simulink model "generic_src"  (Simulink 10.3)
settings: Solver=ode45  StartTime=0.0  StopTime=inf  RelTol=1e-3  EnableMultiTasking=on
undefined symbols (not defined in the file or in its folder): Area_Front, Area_Rear, ay_max_off, ay_max_on, ay_per_mu_max_off, ay_per_mu_max_on, Brake_ratio, brake_valve_ctrl_kP, cat1mode1_higher, cat1mode1_lower, cat1mode2_higher, cat1mode2_lower, cat1mode3_higher, cat1mode3_lower, cat2mode1_higher, cat2mode1_lower, cat2mode2_higher, cat2mode2_lower, cat2mode3_higher, cat2mode3_lower, delta_vel, diff_lock_fac, diff_lock_off, diff_lock_on, ESP_ctrl_kD, ESP_ctrl_kI, ESP_ctrl_kP, ESP_ctrl_restore_kI, ESP_min_throttle_fac, f_ax, f_slip, g, higherlimit_highvel, higherlimit_lowvel, highervel_fac, highervelocity_fac, InitialConditionForIntegrator, limit_acc, limit_selectlow, limit_starting, limit_vdiff, locktime_throttle, lowerlimit_highvel, lowerlimit_lowvel, lowervel_fac, lowervelocity_fac, min_throttle, MPS2KMPH, MSR_ctrl_kD, MSR_ctrl_kI, MSR_ctrl_kP, MSR_min_throttle_fac, PID_kP_sideslip, PID_kP_yawrate, RADpS2RpM, rBrake, RpM2RADpS, SH_SL_switch, sideslip_vel_corr, sidesplip_deviation_max ... (+35)
libraries: CarMaker4SL x137, simulink x57, simulink_extras x6
(part 4 of 12)

== system generic_src/CarMaker/IPG Vehicle/Brake/HydBrakeCU Example/ESP Controller/ESP Input Signals ==
  HydBrakeCtrl_In : Inport
  " " : simulink_extras/Transformations/Radians to Degrees
  "   " : simulink_extras/Transformations/Radians to Degrees
  Bus Creator1 : BusCreator  Inputs=20
  Bus Selector : BusSelector  OutputSignals=Omega_B z,Acc_B y,Acc_B x
  Bus Selector1 : BusSelector  OutputSignals=HydBrakeCU pMC,HydBrakeCU pWB_FL,HydBrakeCU pWB_FR,HydBrakeCU pWB_RL,HydBrakeCU pWB_RR,HydBrakeCU Park,HydBrakeCU Pedal
  Car InertialSensor : CarMaker4SL/Sensors/Inertial Sensor  xname=YRS  xstime=Continuous
  Gain{,6,9..10,12..17} (10 alike) : Gain  SaturateOnIntegerOverflow=on  OutDataTypeStr=Inherit: Same as input  ParamDataTypeStr=Inherit: Same as input
  Gain{1..5,11} (6 alike) : Gain  Gain=RADpS2RpM  SaturateOnIntegerOverflow=on  OutDataTypeStr=Inherit: Same as input  ParamDataTypeStr=Inherit: Same as input
  Gain7 : Gain  Gain=1/g  SaturateOnIntegerOverflow=on  OutDataTypeStr=Inherit: Same as input  ParamDataTypeStr=Inherit: Same as input
  Gain8 : Gain  Gain=1/g  SaturateOnIntegerOverflow=on  OutDataTypeStr=Inherit: Same as input  ParamDataTypeStr=Inherit: Same as input
  Read CM Dict1 : CarMaker4SL/Read CM Dict  xname=Car.WheelSpd_FL  xsync=off  xstime=Continuous
  Read CM Dict10 : CarMaker4SL/Read CM Dict  xname=PT.Clutch.0.rotv_out  xsync=off  xstime=Continuous
  Read CM Dict11 : CarMaker4SL/Read CM Dict  xname=Steer.WhlAng  xsync=off  xstime=Continuous
  Read CM Dict12 : CarMaker4SL/Read CM Dict  xname=PT.Engine.Trq  xsync=off  xstime=Continuous
  Read CM Dict15 : CarMaker4SL/Read CM Dict  xname=PT.GearBox.GearNo  xsync=off  xstime=Continuous
  Read CM Dict2 : CarMaker4SL/Read CM Dict  xname=Car.WheelSpd_FR  xsync=off  xstime=Continuous
  Read CM Dict3 : CarMaker4SL/Read CM Dict  xname=Car.WheelSpd_RL  xsync=off  xstime=Continuous
  Read CM Dict4 : CarMaker4SL/Read CM Dict  xname=Car.WheelSpd_RR  xsync=off  xstime=Continuous
  Read CM Dict7 : CarMaker4SL/Read CM Dict  xname=PT.Engine.rotv  xsync=off  xstime=Continuous
  Read CM Dict9 : CarMaker4SL/Read CM Dict  xname=VC.Gas  xsync=off  xstime=Continuous
  Terminator : Terminator
  ESP Signals : Outport  VectorParamsAs1DForOutWhenUnconnected=off
  wires:
  Gain9/1 -> Bus Creator1/9  "Engine crankshaft output torque [Nm]"
  Gain13/1 -> Bus Creator1/14  "GearState [-]"
  " "/1 -> Bus Creator1/13  "Steering Wheel Angle [deg]"
  Gain11/1 -> Bus Creator1/12  "Torque Converter Speed [rpm]"
  Gain10/1 -> Bus Creator1/10  "Master Cylinder Pressure [bar]"
  Gain8/1 -> Bus Creator1/7  "Sensor Longitudinal acceleration [g]"
  Gain7/1 -> Bus Creator1/6  "Sensor Lateral acceleration [g]"
  "   "/1 -> Bus Creator1/5  "Sensor YawRate [degs]"
  Gain4/1 -> Bus Creator1/4  "WheelSpd RR [rpm]"
  Gain5/1 -> Bus Creator1/3  "WheelSpd RL [rpm]"
  Gain3/1 -> Bus Creator1/2  "WheelSpd FR [rpm]"
  Gain2/1 -> Bus Creator1/1  "WheelSpd FL [rpm]"
  Read CM Dict15/1 -> Gain13/1  "GearNumber [-]"
  Gain1/1 -> Bus Creator1/8  "Engine Speed [rpm]"
  Bus Selector/1 -> "   "/1  "<Omega_B z>"
  Bus Selector/3 -> Gain8/1  "<Acc_B x>"
  Car InertialSensor/2 -> Bus Selector/1
  Read CM Dict11/1 -> " "/1  "Steering Angle [rad]"
  Read CM Dict10/1 -> Gain11/1  "Clucth OutShaft [rad/s]"
  Read CM Dict9/1 -> Gain/1  "Accelerator pedal [-]"
  Bus Selector1/1 -> Gain10/1  "<HydBrakeCU pMC>"
  Read CM Dict1/1 -> Gain2/1  "WheelSpd FL [rad]/s]"
  Read CM Dict2/1 -> Gain3/1  "WheelSpd FR [rad/s]"
  Read CM Dict3/1 -> Gain5/1  "WheelSpd RL [rad/s]"
  Bus Selector/2 -> Gain7/1  "<Acc_B y>"
  Read CM Dict4/1 -> Gain4/1  "WheelSpd RR [rad/s]"
  Gain/1 -> Bus Creator1/11  "Throttle Valve Position"
  Read CM Dict12/1 -> Gain9/1  "Engine Torque [Nm]"
  Read CM Dict7/1 -> Gain1/1  "Engine RotVel [rad/s]"
  Bus Creator1/1 -> ESP Signals/1
  Bus Selector1/5 -> Gain15/1  "<HydBrakeCU pWB_RR>"
  Bus Selector1/4 -> Gain14/1  "<HydBrakeCU pWB_RL>"
  Bus Selector1/3 -> Gain12/1  "<HydBrakeCU pWB_FR>"
  Bus Selector1/2 -> Gain6/1  "<HydBrakeCU pWB_FL>"
  Gain6/1 -> Bus Creator1/15  "Cylinder Pressure FL [bar]"
  Gain12/1 -> Bus Creator1/16  "Cylinder Pressure FR [bar]"
  Gain14/1 -> Bus Creator1/17  "Cylinder Pressure RL [bar]"
  Gain15/1 -> Bus Creator1/18  "Cylinder Pressure RR [bar]"
  HydBrakeCtrl_In/1 -> Bus Selector1/1
  Car InertialSensor/1 -> Terminator/1
  Bus Selector1/6 -> Gain16/1  "<HydBrakeCU Park>"
  Gain16/1 -> Bus Creator1/19  "Park Brake Position"
  Bus Selector1/7 -> Gain17/1  "<HydBrakeCU Pedal>"
  Gain17/1 -> Bus Creator1/20  "Brake Pedal Position"

== system generic_src/CarMaker/IPG Vehicle/Brake/HydBrakeCU Example/ESP Controller/Ideal Input Signals ==
  Bus Creator1 : BusCreator  Inputs=8
  Bus Creator2 : BusCreator  Inputs=4
  Bus Creator3 : BusCreator  Inputs=2
  Bus Creator4 : BusCreator  Inputs=2
  Bus Creator5 : BusCreator  Inputs=3
  Bus Creator6 : BusCreator  Inputs=2
  Read CM Dict1 : CarMaker4SL/Read CM Dict  xname=Car.Pitch  xsync=off  xstime=Continuous
  Read CM Dict10 : CarMaker4SL/Read CM Dict  xname=Car.FzRL  xsync=off  xstime=Continuous
  Read CM Dict11 : CarMaker4SL/Read CM Dict  xname=Car.YawRate  xsync=off  xstime=Continuous
  Read CM Dict13 : CarMaker4SL/Read CM Dict  xname=Car.CRL.Trq_T2W  xsync=off  xstime=Continuous
  Read CM Dict14 : CarMaker4SL/Read CM Dict  xname=Car.LongSlipRL  xsync=off  xstime=Continuous
  Read CM Dict16 : CarMaker4SL/Read CM Dict  xname=Car.CRR.Trq_T2W  xsync=off  xstime=Continuous
  Read CM Dict17 : CarMaker4SL/Read CM Dict  xname=Car.FzRR  xsync=off  xstime=Continuous
  Read CM Dict19 : CarMaker4SL/Read CM Dict  xname=Car.LongSlipRR  xsync=off  xstime=Continuous
  Read CM Dict2 : CarMaker4SL/Read CM Dict  xname=Car.v  xsync=off  xstime=Continuous
  Read CM Dict3 : CarMaker4SL/Read CM Dict  xname=Car.muRoadFR  xsync=off  xstime=Continuous
  Read CM Dict4 : CarMaker4SL/Read CM Dict  xname=Car.muRoadRL  xsync=off  xstime=Continuous
  Read CM Dict5 : CarMaker4SL/Read CM Dict  xname=Car.SideSlipAngle  xsync=off  xstime=Continuous
  Read CM Dict6 : CarMaker4SL/Read CM Dict  xname=Car.muRoadFL  xsync=off  xstime=Continuous
  Read CM Dict7 : CarMaker4SL/Read CM Dict  xname=Car.muRoadRR  xsync=off  xstime=Continuous
  Read CM Dict8 : CarMaker4SL/Read CM Dict  xname=Car.vx  xsync=off  xstime=Continuous
  Read CM Dict9 : CarMaker4SL/Read CM Dict  xname=Car.vy  xsync=off  xstime=Continuous
  Ideal_In : Outport  VectorParamsAs1DForOutWhenUnconnected=off
  wires:
  Read CM Dict17/1 -> Bus Creator4/2  "Ideal_FzRR"
  Read CM Dict10/1 -> Bus Creator4/1  "Ideal_FzRL"
  Read CM Dict16/1 -> Bus Creator3/2  "Ideal_Trq2WRR"
  Read CM Dict13/1 -> Bus Creator3/1  "Ideal_Trq2WRL"
  Read CM Dict6/1 -> Bus Creator2/1  "Ideal_muFL"
  Read CM Dict3/1 -> Bus Creator2/2  "Ideal_muFR"
  Read CM Dict4/1 -> Bus Creator2/3  "Ideal_muRL"
  Read CM Dict7/1 -> Bus Creator2/4  "Ideal_muRR"
  Bus Creator1/1 -> Ideal_In/1
  Read CM Dict1/1 -> Bus Creator1/1  "Ideal_Pitch"
  Read CM Dict5/1 -> Bus Creator1/3  "Ideal_SideSlipAngle"
  Read CM Dict2/1 -> Bus Creator5/1  "Ideal_Velocity"
  Read CM Dict8/1 -> Bus Creator5/2  "Ideal_Velocity_x"
  Bus Creator5/1 -> Bus Creator1/2  "Ideal_Velocity"
  Read CM Dict9/1 -> Bus Creator5/3  "Ideal_Velocity_y"
  Read CM Dict14/1 -> Bus Creator6/1  "Ideal_SlipRL"
  Read CM Dict19/1 -> Bus Creator6/2  "Ideal_SlipRR"
  Read CM Dict11/1 -> Bus Creator1/4  "Ideal_YawRate"
  Bus Creator2/1 -> Bus Creator1/5  "Ideal_mu"
  Bus Creator3/1 -> Bus Creator1/6  "Idea_Trq2W"
  Bus Creator4/1 -> Bus Creator1/7  "Ideal_Fz"
  Bus Creator6/1 -> Bus Creator1/8  "Ideal_Slip"

== system generic_src/CarMaker/IPG Vehicle/Brake/HydBrakeCU Example/ESP Controller/Output Signals ESP ==
  ESP Out : Inport
  Bus Creator : BusCreator  Inputs=6
  Bus Selector : BusSelector  OutputSignals=ECU Flags,Brake Valves,Pilot Valves,Suction Valves,Pump Ctrl,VC_Out.BrakePark,VC_Out.Brake Pedal Position,Diff_Torque,VC_Out.Load_lim
  Bus Selector1 : BusSelector  OutputSignals=ESP On,ASR On,ABS On,HSA On
  Bus Selector2 : BusSelector  OutputSignals=ASR On,MSR On,BMR On
  Bus Selector4 : BusSelector  OutputSignals=FrontDiff_Torque
  Data Type Conversion : DataTypeConversion
  Define CM Dict1 : CarMaker4SL/Define CM Dict  xname=ESP.ASR.MSR.active  xmono=off  xtype=Char  xdvaplace=VC  xnstates=2  xfirststate=0  xinitial=0
  Define CM Dict10 : CarMaker4SL/Define CM Dict  xname=ESP.ESP.active  xmono=off  xtype=Char  xdvaplace=VC  xnstates=2  xfirststate=0  xinitial=0
  Define CM Dict2 : CarMaker4SL/Define CM Dict  xname=ESP.ASR.BMR.active  xmono=off  xtype=Char  xdvaplace=VC  xnstates=2  xfirststate=0  xinitial=0
  Define CM Dict3 : CarMaker4SL/Define CM Dict  xname=ESP.ASR.active  xmono=off  xtype=Char  xdvaplace=VC  xnstates=2  xfirststate=0  xinitial=0
  Define CM Dict4 : CarMaker4SL/Define CM Dict  xname=ESP.HSA.active  xmono=off  xtype=Char  xdvaplace=VC  xnstates=2  xfirststate=0  xinitial=0
  Define CM Dict6 : CarMaker4SL/Define CM Dict  xname=ESP.ESP.lamp  xmono=off  xtype=Char  xdvaplace=VC  xnstates=2  xfirststate=0  xinitial=0
  Define CM Dict9 : CarMaker4SL/Define CM Dict  xname=ESP.ABS.Active  xmono=off  xtype=Char  xdvaplace=VC  xnstates=2  xfirststate=0  xinitial=0
  Logical Operator : Logic  Operator=OR  AllPortsSameDT=off  OutDataTypeStr=boolean
  Read CM Dict3 : CarMaker4SL/Read CM Dict  xname=ESP.User.ESP_off  xsync=off  xstime=Continuous
  Write CM Dict : CarMaker4SL/Write CM Dict  xname=PT.ECU.Load_lim_max  xsync=off
  Write CM Dict12 : CarMaker4SL/Write CM Dict  xname=ESP.ASR.MSR.active  xsync=off
  Write CM Dict13 : CarMaker4SL/Write CM Dict  xname=ESP.ASR.BMR.active  xsync=off
  Write CM Dict15 : CarMaker4SL/Write CM Dict  xname=ESP.ASR.active  xsync=off
  Write CM Dict17 : CarMaker4SL/Write CM Dict  xname=ESP.ABS.Active  xsync=off
  Write CM Dict18 : CarMaker4SL/Write CM Dict  xname=ESP.ESP.active  xsync=off
  Write CM Dict19 : CarMaker4SL/Write CM Dict  xname=PT.Gen.DL.FDiff.DVA.Trq_A2B  xsync=off
  Write CM Dict20 : CarMaker4SL/Write CM Dict  xname=ESP.HSA.active  xsync=off
  Write CM Dict21 : CarMaker4SL/Write CM Dict  xname=ESP.ESP.lamp  xsync=off
  HydBrakeCU_Out : Outport  VectorParamsAs1DForOutWhenUnconnected=off
  wires:
  ESP Out/1 -> Bus Selector/1
  Bus Selector/1 -> Bus Selector1/1  "<ECU Flags>"
  Bus Selector1/2 -> Bus Selector2/1  "<ASR On>"
  Bus Selector1/1 -> Logical Operator/2, Write CM Dict18/1  "<ESP On>"
  Bus Selector1/3 -> Write CM Dict17/1  "<ABS On>"
  Bus Selector2/1 -> Write CM Dict15/1  "<ASR On>"
  Bus Selector2/2 -> Write CM Dict12/1  "<MSR On>"
  Bus Selector2/3 -> Write CM Dict13/1  "<BMR On>"
  Bus Selector4/1 -> Write CM Dict19/1  "<FrontDiff_Torque>"
  Bus Selector/8 -> Bus Selector4/1  "<Diff_Torque>"
  Bus Selector1/4 -> Write CM Dict20/1  "<HSA On>"
  Logical Operator/1 -> Data Type Conversion/1
  Read CM Dict3/1 -> Logical Operator/1
  Data Type Conversion/1 -> Write CM Dict21/1
  Bus Selector/2 -> Bus Creator/1  "<Brake Valves>"
  Bus Selector/3 -> Bus Creator/2  "<Pilot Valves>"
  Bus Selector/4 -> Bus Creator/3  "<Suction Valves>"
  Bus Selector/5 -> Bus Creator/4  "<Pump Ctrl>"
  Bus Creator/1 -> HydBrakeCU_Out/1
  Bus Selector/6 -> Bus Creator/5  "<BrakePark>"
  Bus Selector/9 -> Write CM Dict/1  "<Load_lim>"
  Bus Selector/7 -> Bus Creator/6  "<Brake Pedal Position>"

== system generic_src/CarMaker/IPG Vehicle/Brake/HydBrakeCU Example/ESP Controller/User Input Signals1 ==
  note: User_Drive: 1 = Front; 2 = Rear; 3 = AllWheel
  Bus Creator1 : BusCreator  Inputs=5
  Bus Creator2 : BusCreator  Inputs=5
  Bus Creator3 : BusCreator  Inputs=2
  Bus Creator4 : BusCreator  Inputs=2
  Define CM Dict1 : CarMaker4SL/Define CM Dict  xname=ESP.User.ESP_off  xmono=off  xtype=Char  xdvaplace=IO_Out  xnstates=2  xfirststate=0  xinitial=0
  Define CM Dict10 : CarMaker4SL/Define CM Dict  xname=ESP.User.HSA_off  xmono=off  xtype=Char  xdvaplace=IO_Out  xnstates=2  xfirststate=0  xinitial=0
  Define CM Dict11 : CarMaker4SL/Define CM Dict  xname=ESP.User.oneWheel_on  xmono=off  xtype=Char  xdvaplace=IO_Out  xnstates=2  xfirststate=0  xinitial=0
  Define CM Dict2 : CarMaker4SL/Define CM Dict  xname=ESP.User.ASR_off  xmono=off  xtype=Char  xdvaplace=IO_Out  xnstates=2  xfirststate=0  xinitial=0
  Define CM Dict3 : CarMaker4SL/Define CM Dict  xname=ESP.User.ABS_off  xmono=off  xtype=Char  xdvaplace=IO_Out  xnstates=2  xfirststate=0  xinitial=0
  Define CM Dict4 : CarMaker4SL/Define CM Dict  xname=ESP.User.ESP_all_off  xmono=off  xtype=Char  xdvaplace=IO_Out  xnstates=2  xfirststate=0  xinitial=0
  Define CM Dict5 : CarMaker4SL/Define CM Dict  xname=ESP.User.Drive  xmono=off  xtype=Char  xdvaplace=IO_Out  xnstates=3  xfirststate=1  xinitial=1
  Define CM Dict6 : CarMaker4SL/Define CM Dict  xname=ESP.User.SideSlip_estimator_on  xmono=off  xtype=Char  xdvaplace=IO_Out  xnstates=2  xfirststate=0  xinitial=0
  Define CM Dict7 : CarMaker4SL/Define CM Dict  xname=ESP.User.mue_estimator_on  xmono=off  xtype=Char  xdvaplace=IO_Out  xnstates=2  xfirststate=0  xinitial=0
  Define CM Dict8 : CarMaker4SL/Define CM Dict  xname=ESP.User.DiffLockDVA_on  xmono=off  xtype=Char  xdvaplace=IO_Out  xnstates=2  xfirststate=0  xinitial=0
  Define CM Dict9 : CarMaker4SL/Define CM Dict  xname=ESP.User.DiffLockDVA_Trq  xunit=Nm  xmono=off  xtype=Double4  xdvaplace=IO_Out  xnstates=2  xfirststate=0  xinitial=0
  Read CM Dict1 : CarMaker4SL/Read CM Dict  xname=ESP.User.Drive  xsync=off  xstime=Continuous
  Read CM Dict10 : CarMaker4SL/Read CM Dict  xname=ESP.User.HSA_off  xsync=off  xstime=Continuous
  Read CM Dict11 : CarMaker4SL/Read CM Dict  xname=ESP.User.oneWheel_on  xsync=off  xstime=Continuous
  Read CM Dict2 : CarMaker4SL/Read CM Dict  xname=ESP.User.ESP_all_off  xsync=off  xstime=Continuous
  Read CM Dict3 : CarMaker4SL/Read CM Dict  xname=ESP.User.ESP_off  xsync=off  xstime=Continuous
  Read CM Dict4 : CarMaker4SL/Read CM Dict  xname=ESP.User.ASR_off  xsync=off  xstime=Continuous
  Read CM Dict5 : CarMaker4SL/Read CM Dict  xname=ESP.User.ABS_off  xsync=off  xstime=Continuous
  Read CM Dict6 : CarMaker4SL/Read CM Dict  xname=ESP.User.SideSlip_estimator_on  xsync=off  xstime=Continuous
  Read CM Dict7 : CarMaker4SL/Read CM Dict  xname=ESP.User.mue_estimator_on  xsync=off  xstime=Continuous
  Read CM Dict8 : CarMaker4SL/Read CM Dict  xname=ESP.User.DiffLockDVA_on  xsync=off  xstime=Continuous
  Read CM Dict9 : CarMaker4SL/Read CM Dict  xname=ESP.User.DiffLockDVA_Trq  xsync=off  xstime=Continuous
  User_In : Outport  VectorParamsAs1DForOutWhenUnconnected=off
  wires:
  Read CM Dict1/1 -> Bus Creator1/1  "User_Drive"
  Bus Creator1/1 -> User_In/1
  Read CM Dict5/1 -> Bus Creator2/4  "User_Switch_ABS_off"
  Read CM Dict4/1 -> Bus Creator2/3  "User_Switch_ASR_off"
  Read CM Dict3/1 -> Bus Creator2/2  "User_Switch_ESP_off"
  Read CM Dict2/1 -> Bus Creator2/1  "User_Switch_Main_off"
  Bus Creator2/1 -> Bus Creator1/2  "User_Switch"
  Read CM Dict6/1 -> Bus Creator3/1  "User_SideSlip_estimator_on"
  Read CM Dict7/1 -> Bus Creator3/2  "User_mue_estimator_on"
  Bus Creator3/1 -> Bus Creator1/3  "User_estimators_on"
  Read CM Dict8/1 -> Bus Creator4/1  "User_DiffLock_on"
  Read CM Dict9/1 -> Bus Creator4/2  "User_DiffLock_Trq"
  Bus Creator4/1 -> Bus Creator1/4  "User_DiffLock"
  Read CM Dict10/1 -> Bus Creator2/5  "User_Switch_HSA_off"
  Read CM Dict11/1 -> Bus Creator1/5  "User_oneWheel_on"

== system generic_src/CarMaker/IPG Vehicle/Brake/HydBrakeCU Example/ESP Controller/Vehicle Input Parameter ==
  note: Note:
      | We could also use
      | the left wheel as is has
      | the same coordinate
      | as regards x-axis
      | (which interests us here)
  note: Note:
      | We could also use
      | the left wheel as is has
      | the same coordinate
      | as regards x-axis
      | (which interests us here)
  Bus Creator{,1..3} (4 alike) : BusCreator  Inputs=4
  Bus Creator4 : BusCreator  Inputs=2
  Read CM Parameter : CarMaker4SL/Read CM Parameter  xfile=TireFL  xkey=KinRollRadius  xnout=1  xdefaults=0  xmuxed=on  xstime=Continuous
  Read CM Parameter1 : CarMaker4SL/Read CM Parameter  xfile=TireFR  xkey=KinRollRadius  xnout=1  xdefaults=0  xmuxed=on  xstime=Continuous
  Read CM Parameter2 : CarMaker4SL/Read CM Parameter  xfile=TireRL  xkey=KinRollRadius  xnout=1  xdefaults=0  xmuxed=on  xstime=Continuous
  Read CM Parameter3 : CarMaker4SL/Read CM Parameter  xfile=TireRR  xkey=KinRollRadius  xnout=1  xdefaults=0  xmuxed=on  xstime=Continuous
  Read CM Parameter4 : CarMaker4SL/Read CM Parameter  xfile=Vehicle  xkey=WheelCarrier.fr.pos  xnout=1  xdefaults=0  xmuxed=on  xstime=Continuous
  Read CM Parameter5 : CarMaker4SL/Read CM Parameter  xfile=Vehicle  xkey=Body.pos  xnout=1  xdefaults=0  xmuxed=on  xstime=Continuous
  Read CM Parameter6 : CarMaker4SL/Read CM Parameter  xfile=Vehicle  xkey=Body.pos  xnout=1  xdefaults=0  xmuxed=on  xstime=Continuous
  Read CM Parameter7 : CarMaker4SL/Read CM Parameter  xfile=Vehicle  xkey=WheelCarrier.rr.pos  xnout=1  xdefaults=0  xmuxed=on  xstime=Continuous
  Read CM Parameter8 : CarMaker4SL/Read CM Parameter  xfile=Vehicle  xkey=WheelCarrier.rl.pos  xnout=2  xdefaults=0  xmuxed=off  xstime=Continuous
  Read CM Parameter9 : CarMaker4SL/Read CM Parameter  xfile=Vehicle  xkey=WheelCarrier.fl.pos  xnout=2  xdefaults=0  xmuxed=off  xstime=Continuous
  Steer Angle y-Data : Constant  Value=SteerAng_Out
  Steer Wheel Angle x-Data : Constant  Value=SteerWheelAng_In
  Sum3 : Sum  Inputs=+-  InputSameDT=on  SaturateOnIntegerOverflow=on  OutDataTypeStr=Inherit: Same as first input
  Sum4 : Sum  Inputs=+-  InputSameDT=on  SaturateOnIntegerOverflow=on  OutDataTypeStr=Inherit: Same as first input
  Terminator{,1..9} (10 alike) : Terminator
  z-Position of WheelCarrier FL : CarMaker4SL/Read CM Parameter  xfile=Vehicle  xkey=WheelCarrier.fl.pos  xnout=3  xdefaults=0  xmuxed=off  xstime=Continuous
  z-Position of WheelCarrier FR : CarMaker4SL/Read CM Parameter  xfile=Vehicle  xkey=WheelCarrier.fr.pos  xnout=3  xdefaults=0  xmuxed=off  xstime=Continuous
  z-Position of WheelCarrier RL : CarMaker4SL/Read CM Parameter  xfile=Vehicle  xkey=WheelCarrier.rl.pos  xnout=3  xdefaults=0  xmuxed=off  xstime=Continuous
  z-Position of WheelCarrier RR : CarMaker4SL/Read CM Parameter  xfile=Vehicle  xkey=WheelCarrier.rr.pos  xnout=3  xdefaults=0  xmuxed=off  xstime=Continuous
  Vehicle Param : Outport  VectorParamsAs1DForOutWhenUnconnected=off
  wires:
  Bus Creator1/1 -> Vehicle Param/1
  Read CM Parameter1/1 -> Bus Creator/2  "Param_RadiusFR"
  Read CM Parameter3/1 -> Bus Creator/4  "Param_RadiusRR"
  Bus Creator/1 -> Bus Creator1/1  "TireRadius"
  Read CM Parameter/1 -> Bus Creator/1  "Param_RadiusFL"
  Read CM Parameter2/1 -> Bus Creator/3  "Param_RadiusRL"
  Read CM Parameter5/1 -> Sum4/2
  Read CM Parameter4/1 -> Sum4/1
  Sum4/1 -> Bus Creator2/1  "Param_aF"
  Read CM Parameter7/1 -> Sum3/2
  Sum3/1 -> Bus Creator2/2  "Param_aR"
  Read CM Parameter6/1 -> Sum3/1
  Bus Creator2/1 -> Bus Creator1/2  "VehicleGeometry"
  Read CM Parameter8/2 -> Bus Creator2/4  "Param_bR"
  Read CM Parameter9/2 -> Bus Creator2/3  "Param_bF"
  Read CM Parameter9/1 -> Terminator/1
  Read CM Parameter8/1 -> Terminator1/1
  z-Position of WheelCarrier FL/1 -> Terminator2/1
  z-Position of WheelCarrier FL/2 -> Terminator3/1
  Bus Creator3/1 -> Bus Creator1/3  "CarrierGeometry"
  z-Position of WheelCarrier FL/3 -> Bus Creator3/1  "Param_zFL"
  z-Position of WheelCarrier FR/3 -> Bus Creator3/2  "Param_zFR"
  z-Position of WheelCarrier RL/3 -> Bus Creator3/3  "Param_zRL"
  z-Position of WheelCarrier RR/3 -> Bus Creator3/4  "Param_zRR"
  z-Position of WheelCarrier FR/1 -> Terminator4/1
  z-Position of WheelCarrier FR/2 -> Terminator5/1
  z-Position of WheelCarrier RL/1 -> Terminator6/1
  z-Position of WheelCarrier RL/2 -> Terminator7/1
  z-Position of WheelCarrier RR/1 -> Terminator8/1
  z-Position of WheelCarrier RR/2 -> Terminator9/1
  Steer Angle y-Data/1 -> Bus Creator4/2  "SteerAng_Out"
  Steer Wheel Angle x-Data/1 -> Bus Creator4/1  "SteerWheelAng_In"
  Bus Creator4/1 -> Bus Creator1/4  "SteeringGeometry"

== system generic_src/CarMaker/IPG Vehicle/Brake/HydBrakeCU Example/HydBrakeCtrl_In/CreateBus HydBrakeCU ==
  In : Inport
  BusCreator : BusCreator  Inputs=45
  Demux : Demux  Outputs=45
      settings: DisplayOption=none
  Ground{,1..14} (15 alike) : Ground
  Terminator{,1..14} (15 alike) : Terminator
  Out : Outport  VectorParamsAs1DForOutWhenUnconnected=off
  wires:
  In/1 -> Demux/1
  BusCreator/1 -> Out/1
  Demux/1 -> BusCreator/1  "HydBrakeCU Pedal"
  Demux/2 -> BusCreator/2  "HydBrakeCU Park"
  Demux/3 -> BusCreator/3  "HydBrakeCU Trq_BrakeReg_max_FL"
  Demux/4 -> BusCreator/4  "HydBrakeCU Trq_BrakeReg_max_FR"
  Demux/5 -> BusCreator/5  "HydBrakeCU Trq_BrakeReg_max_RL"
  Demux/6 -> BusCreator/6  "HydBrakeCU Trq_BrakeReg_max_RR"
  Demux/7 -> BusCreator/7  "HydBrakeCU Trq_BrakeReg_FL"
  Demux/8 -> BusCreator/8  "HydBrakeCU Trq_BrakeReg_FR"
  Demux/9 -> BusCreator/9  "HydBrakeCU Trq_BrakeReg_RL"
  Demux/10 -> BusCreator/10  "HydBrakeCU Trq_BrakeReg_RR"
  Demux/11 -> BusCreator/11  "HydBrakeCU T_env"
  Demux/12 -> BusCreator/12  "HydBrakeCU Trq_WB_FL"
  Demux/13 -> BusCreator/13  "HydBrakeCU Trq_WB_FR"
  Demux/14 -> BusCreator/14  "HydBrakeCU Trq_WB_RL"
  Demux/15 -> BusCreator/15  "HydBrakeCU Trq_WB_RR"
  Demux/16 -> BusCreator/16  "HydBrakeCU Trq_PB_FL"
  Demux/17 -> BusCreator/17  "HydBrakeCU Trq_PB_FR"
  Demux/18 -> BusCreator/18  "HydBrakeCU Trq_PB_RL"
  Demux/19 -> BusCreator/19  "HydBrakeCU Trq_PB_RR"
  Demux/20 -> BusCreator/20  "HydBrakeCU Rel_SW"
  Demux/21 -> BusCreator/21  "HydBrakeCU pMC"
  Demux/22 -> BusCreator/22
  Demux/23 -> Terminator14/1  "HydBrakeCU pWB_FL"
  Demux/24 -> BusCreator/24  "HydBrakeCU pWB_FR"
  Demux/25 -> BusCreator/25  "HydBrakeCU pWB_RL"
  Demux/26 -> BusCreator/26  "HydBrakeCU pWB_RR"
  Demux/27 -> BusCreator/27  "HydBrakeCU PuRetVolt"
  Demux/28 -> BusCreator/28  "HydBrakeCU PedFrc"
  Demux/29 -> BusCreator/29  "HydBrakeCU PedTravel"
  Demux/30 -> BusCreator/30  "HydBrakeCU PistTravel"
  Demux/45 -> Terminator/1
  Demux/44 -> Terminator1/1
  Demux/43 -> Terminator2/1
  Demux/42 -> Terminator3/1
  Demux/41 -> Terminator4/1
  Demux/40 -> Terminator5/1
  Demux/39 -> Terminator6/1
  Demux/38 -> Terminator7/1
  Demux/37 -> Terminator8/1
  Demux/36 -> Terminator9/1
  Demux/35 -> Terminator10/1
  Demux/34 -> Terminator11/1
  Demux/33 -> Terminator12/1
  Demux/32 -> Terminator13/1
  Ground/1 -> BusCreator/45
  Ground1/1 -> BusCreator/44
  Ground2/1 -> BusCreator/43
  Ground3/1 -> BusCreator/42
  Ground4/1 -> BusCreator/41
  Ground5/1 -> BusCreator/40
  Ground6/1 -> BusCreator/39
  Ground7/1 -> BusCreator/38
  Ground8/1 -> BusCreator/37
  Ground9/1 -> BusCreator/36
  Ground10/1 -> BusCreator/35
  Ground11/1 -> BusCreator/34
  Ground12/1 -> BusCreator/33
  Ground13/1 -> BusCreator/32
  Demux/31 -> BusCreator/31  "HydBrakeCU DiaphTravel"
  Ground14/1 -> BusCreator/23

== system generic_src/CarMaker/IPG Vehicle/Brake/HydBrakeCU Example/HydBrakeCtrl_In/CreateBus HydBrakeCU_Cfg ==
  In : Inport
  BusCreator : BusCreator  Inputs=4
  Demux : Demux
      settings: DisplayOption=none
  Ground : Ground
  Terminator : Terminator
  Out : Outport  VectorParamsAs1DForOutWhenUnconnected=off
  wires:
  In/1 -> Demux/1
  BusCreator/1 -> Out/1
  Demux/1 -> BusCreator/1  "HydBrakeCU_Cfg VhclClassId"
  Demux/2 -> BusCreator/2  "HydBrakeCU_Cfg nWheels"
  Demux/3 -> BusCreator/3  "HydBrakeCU_Cfg BrakeKind"
  Ground/1 -> BusCreator/4
  Demux/4 -> Terminator/1

== system generic_src/CarMaker/IPG Vehicle/CarAndTrailer/Forces/Tires/TireFL ==
  note: Insert your tire model here.
  Sync_In : Inport
  Load : Inport  Port=2
  vxtrans : Inport  Port=3
  vytrans : Inport  Port=4
  Rim_rotv : Inport  Port=5
  Rim_turnv : Inport  Port=6
  InclinAngle : Inport  Port=7
  muRoad : Inport  Port=8
  Ground{1..11} (11 alike) : Ground
  Terminator{,1..6,12} (8 alike) : Terminator
  Slp : Outport  VectorParamsAs1DForOutWhenUnconnected=off
  Alpha : Outport  Port=2  VectorParamsAs1DForOutWhenUnconnected=off
  TurnSlp : Outport  Port=3  VectorParamsAs1DForOutWhenUnconnected=off
  rBelt_eff : Outport  Port=4  VectorParamsAs1DForOutWhenUnconnected=off
  vBelt : Outport  Port=5  VectorParamsAs1DForOutWhenUnconnected=off
  LongFrc : Outport  Port=6  VectorParamsAs1DForOutWhenUnconnected=off
  SideFrc : Outport  Port=7  VectorParamsAs1DForOutWhenUnconnected=off
  LoadFrc : Outport  Port=8  VectorParamsAs1DForOutWhenUnconnected=off
  OverturnTrq : Outport  Port=9  VectorParamsAs1DForOutWhenUnconnected=off
  RollResist : Outport  Port=10  VectorParamsAs1DForOutWhenUnconnected=off
  AlignTrq : Outport  Port=11  VectorParamsAs1DForOutWhenUnconnected=off
  wires:
  Ground11/1 -> vBelt/1
  Ground10/1 -> rBelt_eff/1
  Ground9/1 -> TurnSlp/1
  Rim_turnv/1 -> Terminator6/1
  Sync_In/1 -> Terminator12/1
  Ground2/1 -> Alpha/1
  Ground3/1 -> LongFrc/1
  Ground4/1 -> SideFrc/1
  Ground5/1 -> OverturnTrq/1
  vxtrans/1 -> Terminator1/1
  vytrans/1 -> Terminator2/1
  Rim_rotv/1 -> Terminator3/1
  InclinAngle/1 -> Terminator4/1
  muRoad/1 -> Terminator5/1
  Load/1 -> Terminator/1
  Ground1/1 -> Slp/1
  Ground6/1 -> LoadFrc/1
  Ground7/1 -> RollResist/1
  Ground8/1 -> AlignTrq/1

== system generic_src/CarMaker/IPG Vehicle/CarAndTrailer/Forces/Tires/TireFR ==
  note: Insert your tire model here.
  Sync_In : Inport
  Load : Inport  Port=2
  vxtrans : Inport  Port=3
  vytrans : Inport  Port=4
  Rim_rotv : Inport  Port=5
  Rim_turnv : Inport  Port=6
  InclinAngle : Inport  Port=7
  muRoad : Inport  Port=8
  Ground{1..11} (11 alike) : Ground
  Terminator{,1..6,12} (8 alike) : Terminator
  Slp : Outport  VectorParamsAs1DForOutWhenUnconnected=off
  Alpha : Outport  Port=2  VectorParamsAs1DForOutWhenUnconnected=off
  TurnSlp : Outport  Port=3  VectorParamsAs1DForOutWhenUnconnected=off
  rBelt_eff : Outport  Port=4  VectorParamsAs1DForOutWhenUnconnected=off
  vBelt : Outport  Port=5  VectorParamsAs1DForOutWhenUnconnected=off
  LongFrc : Outport  Port=6  VectorParamsAs1DForOutWhenUnconnected=off
  SideFrc : Outport  Port=7  VectorParamsAs1DForOutWhenUnconnected=off
  LoadFrc : Outport  Port=8  VectorParamsAs1DForOutWhenUnconnected=off
  OverturnTrq : Outport  Port=9  VectorParamsAs1DForOutWhenUnconnected=off
  RollResist : Outport  Port=10  VectorParamsAs1DForOutWhenUnconnected=off
  AlignTrq : Outport  Port=11  VectorParamsAs1DForOutWhenUnconnected=off
  wires:
  Ground11/1 -> vBelt/1
  Ground10/1 -> rBelt_eff/1
  Ground9/1 -> TurnSlp/1
  Rim_turnv/1 -> Terminator6/1
  Sync_In/1 -> Terminator12/1
  Ground2/1 -> Alpha/1
  Ground3/1 -> LongFrc/1
  Ground4/1 -> SideFrc/1
  Ground5/1 -> OverturnTrq/1
  vxtrans/1 -> Terminator1/1
  vytrans/1 -> Terminator2/1
  Rim_rotv/1 -> Terminator3/1
  InclinAngle/1 -> Terminator4/1
  muRoad/1 -> Terminator5/1
  Load/1 -> Terminator/1
  Ground1/1 -> Slp/1
  Ground6/1 -> LoadFrc/1
  Ground7/1 -> RollResist/1
  Ground8/1 -> AlignTrq/1

== system generic_src/CarMaker/IPG Vehicle/CarAndTrailer/Forces/Tires/TireRL ==
  note: Insert your tire model here.
  Sync_In : Inport
  Load : Inport  Port=2
  vxtrans : Inport  Port=3
  vytrans : Inport  Port=4
  Rim_rotv : Inport  Port=5
  Rim_turnv : Inport  Port=6
  InclinAngle : Inport  Port=7
  muRoad : Inport  Port=8
  Ground{1..11} (11 alike) : Ground
  Terminator{,1..6,12} (8 alike) : Terminator
  Slp : Outport  VectorParamsAs1DForOutWhenUnconnected=off
  Alpha : Outport  Port=2  VectorParamsAs1DForOutWhenUnconnected=off
  TurnSlp : Outport  Port=3  VectorParamsAs1DForOutWhenUnconnected=off
  rBelt_eff : Outport  Port=4  VectorParamsAs1DForOutWhenUnconnected=off
  vBelt : Outport  Port=5  VectorParamsAs1DForOutWhenUnconnected=off
  LongFrc : Outport  Port=6  VectorParamsAs1DForOutWhenUnconnected=off
  SideFrc : Outport  Port=7  VectorParamsAs1DForOutWhenUnconnected=off
  LoadFrc : Outport  Port=8  VectorParamsAs1DForOutWhenUnconnected=off
  OverturnTrq : Outport  Port=9  VectorParamsAs1DForOutWhenUnconnected=off
  RollResist : Outport  Port=10  VectorParamsAs1DForOutWhenUnconnected=off
  AlignTrq : Outport  Port=11  VectorParamsAs1DForOutWhenUnconnected=off
  wires:
  Ground11/1 -> vBelt/1
  Ground10/1 -> rBelt_eff/1
  Ground9/1 -> TurnSlp/1
  Rim_turnv/1 -> Terminator6/1
  Sync_In/1 -> Terminator12/1
  Ground2/1 -> Alpha/1
  Ground3/1 -> LongFrc/1
  Ground4/1 -> SideFrc/1
  Ground5/1 -> OverturnTrq/1
  vxtrans/1 -> Terminator1/1
  vytrans/1 -> Terminator2/1
  Rim_rotv/1 -> Terminator3/1
  InclinAngle/1 -> Terminator4/1
  muRoad/1 -> Terminator5/1
  Load/1 -> Terminator/1
  Ground1/1 -> Slp/1
  Ground6/1 -> LoadFrc/1
  Ground7/1 -> RollResist/1
  Ground8/1 -> AlignTrq/1

== system generic_src/CarMaker/IPG Vehicle/CarAndTrailer/Forces/Tires/TireRR ==
  note: Insert your tire model here.
  Sync_In : Inport
  Load : Inport  Port=2
  vxtrans : Inport  Port=3
  vytrans : Inport  Port=4
  Rim_rotv : Inport  Port=5
  Rim_turnv : Inport  Port=6
  InclinAngle : Inport  Port=7
  muRoad : Inport  Port=8
  Ground{1..11} (11 alike) : Ground
  Terminator{,1..6,12} (8 alike) : Terminator
  Slp : Outport  VectorParamsAs1DForOutWhenUnconnected=off
  Alpha : Outport  Port=2  VectorParamsAs1DForOutWhenUnconnected=off
  TurnSlp : Outport  Port=3  VectorParamsAs1DForOutWhenUnconnected=off
  rBelt_eff : Outport  Port=4  VectorParamsAs1DForOutWhenUnconnected=off
  vBelt : Outport  Port=5  VectorParamsAs1DForOutWhenUnconnected=off
  LongFrc : Outport  Port=6  VectorParamsAs1DForOutWhenUnconnected=off
  SideFrc : Outport  Port=7  VectorParamsAs1DForOutWhenUnconnected=off
  LoadFrc : Outport  Port=8  VectorParamsAs1DForOutWhenUnconnected=off
  OverturnTrq : Outport  Port=9  VectorParamsAs1DForOutWhenUnconnected=off
  RollResist : Outport  Port=10  VectorParamsAs1DForOutWhenUnconnected=off
  AlignTrq : Outport  Port=11  VectorParamsAs1DForOutWhenUnconnected=off
  wires:
  Ground11/1 -> vBelt/1
  Ground10/1 -> rBelt_eff/1
  Ground9/1 -> TurnSlp/1
  Rim_turnv/1 -> Terminator6/1
  Sync_In/1 -> Terminator12/1
  Ground2/1 -> Alpha/1
  Ground3/1 -> LongFrc/1
  Ground4/1 -> SideFrc/1
  Ground5/1 -> OverturnTrq/1
  vxtrans/1 -> Terminator1/1
  vytrans/1 -> Terminator2/1
  Rim_rotv/1 -> Terminator3/1
  InclinAngle/1 -> Terminator4/1
  muRoad/1 -> Terminator5/1
  Load/1 -> Terminator/1
  Ground1/1 -> Slp/1
  Ground6/1 -> LoadFrc/1
  Ground7/1 -> RollResist/1
  Ground8/1 -> AlignTrq/1

== system generic_src/CarMaker/IPG Vehicle/PowerTrain/MCU Example/MyMotorCU/Enabled Subsystem ==
  rotv : Inport
  Trq_trg : Inport  Port=2
  Load : Inport  Port=3
  rotv_trg : Inport  Port=4
  Ratio : Inport  Port=5
  TrqMot_max table : Inport  Port=6
  TrqGen_max table : Inport  Port=7
  rotv_Mot_max : Inport  Port=8
  rotv_Gen_max : Inport  Port=9
  Enable : EnablePort
  Abs : Abs
  Abs1 : Abs
  Abs2 : Abs
  Bus Selector : BusSelector  OutputSignals=x,z
  Bus Selector1 : BusSelector  OutputSignals=x,z
  Compare To Constant : simulink/Logic and Bit Operations/Compare To Constant  relop===  const=-99999  OutDataTypeStr=uint8  ZeroCross=off
  Constant : Constant  Value=0.0
  Constant1 : Constant  Value=0.0
  Gain : Gain  Gain=-1
  Lookup Table Dynamic : simulink/Lookup Tables/Lookup Table Dynamic  LookUpMeth=Interpolation-Use End Values  OutDataType=float('double')  OutScaling=[]  OutputDataTypeScalingMode=Specify via dialog  OutDataTypeStr=float('double')  DoSatur=off
  Lookup Table Dynamic1 : simulink/Lookup Tables/Lookup Table Dynamic  LookUpMeth=Interpolation-Use End Values  OutDataType=float('double')  OutScaling=[]  OutputDataTypeScalingMode=Specify via dialog  OutDataTypeStr=float('double')  DoSatur=off
  MotMode : Subsystem
  Product : Product  RndMeth=Zero
  Product1 : Product  RndMeth=Zero
  Product2 : Product  RndMeth=Zero
  Saturation : Saturate  UpperLimit=1  LowerLimit=-1
  Switch : Switch  Criteria=u2 ~= 0
  Switch1 : Switch  Criteria=u2 ~= 0
  Switch2 : Switch  Criteria=u2 ~= 0
  if condition : Subsystem
  rotv Copy : InportShadow
  Load out : Outport  VectorParamsAs1DForOutWhenUnconnected=off
  TrqMot_max : Outport  Port=2  VectorParamsAs1DForOutWhenUnconnected=off
  TrqGen_max : Outport  Port=3  VectorParamsAs1DForOutWhenUnconnected=off
  wires:
  rotv Copy/1 -> if condition/2(rotv)
  Bus Selector/2 -> Lookup Table Dynamic/3  "<z>"
  Lookup Table Dynamic/1 -> Product1/2
  Abs2/1 -> Switch/1
  Abs1/1 -> Switch/3
  Product/1 -> Lookup Table Dynamic1/1, Lookup Table Dynamic/1  "rotv"
  rotv_trg/1 -> if condition/1(rotv_trg)
  if condition/1(Boolean) -> Switch2/2
  Switch1/1 -> Switch2/3  "Load"
  Constant1/1 -> Switch2/1
  Switch2/1 -> Load out/1
  Saturation/1 -> Switch1/3
  Constant/1 -> Switch1/1
  Compare To Constant/1 -> Switch1/2
  Load/1 -> Saturation/1, Compare To Constant/1
  Trq_trg/1 -> MotMode/1(Trq_trg)
  MotMode/1(Boolean) -> Switch/2
  Gain/1 -> Product2/2
  Product2/1 -> TrqGen_max/1
  Product1/1 -> TrqMot_max/1
  Switch/1 -> if condition/3(lim_rotv)  "lim_rotv"
  rotv_Mot_max/1 -> Abs2/1
  rotv_Gen_max/1 -> Abs1/1
  Lookup Table Dynamic1/1 -> Gain/1
  Bus Selector1/2 -> Lookup Table Dynamic1/3  "<z>"
  Bus Selector1/1 -> Lookup Table Dynamic1/2  "<x>"
  TrqGen_max table/1 -> Bus Selector1/1
  Bus Selector/1 -> Lookup Table Dynamic/2  "<x>"
  TrqMot_max table/1 -> Bus Selector/1
  Abs/1 -> Product/1
  Ratio/1 -> Product1/1, Product2/1, Product/2
  rotv/1 -> MotMode/2(rotv), Abs/1

== system generic_src/CarMaker/IPG Vehicle/PowerTrain/MCU Example/MyMotorCU/ReturnZero ==
  Enable : EnablePort
  Bus Creator : BusCreator  Inputs=3
  Constant : Constant  Value=0.0
  Constant1 : Constant  Value=0.0
  Constant2 : Constant  Value=0.0
  Signal Conversion : SignalConversion  ConversionOutput=Bus copy  OverrideOpt=off
  ReturnZero : Outport  VectorParamsAs1DForOutWhenUnconnected=off
  wires:
  Signal Conversion/1 -> ReturnZero/1
  Constant2/1 -> Bus Creator/3  "TrqGen_max"
  Constant1/1 -> Bus Creator/2  "TrqMot_max"
  Constant/1 -> Bus Creator/1  "Load"
  Bus Creator/1 -> Signal Conversion/1

== system generic_src/CarMaker/IPG Vehicle/PowerTrain/MCU Example/PTMotorCU_In/CreateBus MCU ISGIn ==
  In : Inport
  BusCreator : BusCreator  Inputs=12
  Demux : Demux  Outputs=12
      settings: DisplayOption=none
  Out : Outport  VectorParamsAs1DForOutWhenUnconnected=off
  wires:
  Demux/6 -> BusCreator/6  "MCU ISGIn PwrElec"
  Demux/4 -> BusCreator/4  "MCU ISGIn rotv"
  Demux/3 -> BusCreator/3  "MCU ISGIn rotv_trg"
  Demux/2 -> BusCreator/2  "MCU ISGIn Trq"
  Demux/8 -> BusCreator/8  "MCU ISGIn Current_d"
  Demux/9 -> BusCreator/9  "MCU ISGIn Current_q"
  In/1 -> Demux/1
  Demux/7 -> BusCreator/7  "MCU ISGIn VoltBatt"
  BusCreator/1 -> Out/1
  Demux/1 -> BusCreator/1  "MCU ISGIn Trq_trg"
  Demux/5 -> BusCreator/5  "MCU ISGIn rot"
  Demux/10 -> BusCreator/10  "MCU ISGIn Current_u"
  Demux/11 -> BusCreator/11  "MCU ISGIn Current_v"
  Demux/12 -> BusCreator/12  "MCU ISGIn Current_w"

== system generic_src/CarMaker/IPG Vehicle/PowerTrain/MCU Example/PTMotorCU_In/CreateBus MCU ISGOut ==
  In : Inport
  BusCreator : BusCreator  Inputs=1
  Demux : Demux  Outputs=1
      settings: DisplayOption=none
  Out : Outport  VectorParamsAs1DForOutWhenUnconnected=off
  wires:
  Demux/1 -> BusCreator/1  "MCU ISGIn Load"
  BusCreator/1 -> Out/1
  In/1 -> Demux/1

== system generic_src/CarMaker/IPG Vehicle/PowerTrain/MCU Example/PTMotorCU_In/CreateBus MCU Ignition ==
  In : Inport
  BusCreator : BusCreator  Inputs=1
  Demux : Demux  Outputs=1
      settings: DisplayOption=none
  Out : Outport  VectorParamsAs1DForOutWhenUnconnected=off
  wires:
  Demux/1 -> BusCreator/1  "MCU Ignition"
  BusCreator/1 -> Out/1
  In/1 -> Demux/1

== system generic_src/CarMaker/IPG Vehicle/PowerTrain/MCU Example/PTMotorCU_In/CreateBus MCU MotorIn0 ==
  In : Inport
  BusCreator1 : BusCreator  Inputs=12
  Demux1 : Demux  Outputs=12
      settings: DisplayOption=none
  Out : Outport  VectorParamsAs1DForOutWhenUnconnected=off
  wires:
  In/1 -> Demux1/1
  Demux1/12 -> BusCreator1/12  "MCU MotorIn0 Current_w"
  Demux1/10 -> BusCreator1/10  "MCU MotorIn0 Current_u"
  Demux1/6 -> BusCreator1/6  "MCU MotorIn0 PwrElec"
  Demux1/7 -> BusCreator1/7  "MCU MotorIn0 VoltBatt"
  Demux1/9 -> BusCreator1/9  "MCU MotorIn0 Current_q"
  Demux1/1 -> BusCreator1/1  "MCU MotorIn0 Trq_trg"
  Demux1/3 -> BusCreator1/3  "MCU MotorIn0 rotv_trg"
  BusCreator1/1 -> Out/1
  Demux1/2 -> BusCreator1/2  "MCU MotorIn0 Trq"
  Demux1/4 -> BusCreator1/4  "MCU MotorIn0 rotv"
  Demux1/11 -> BusCreator1/11  "MCU MotorIn0 Current_v"
  Demux1/8 -> BusCreator1/8  "MCU MotorIn0 Current_d"
  Demux1/5 -> BusCreator1/5  "MCU MotorIn0 rot"

== system generic_src/CarMaker/IPG Vehicle/PowerTrain/MCU Example/PTMotorCU_In/CreateBus MCU MotorIn1 ==
  In : Inport
  BusCreator1 : BusCreator  Inputs=12
  Demux1 : Demux  Outputs=12
      settings: DisplayOption=none
  Out : Outport  VectorParamsAs1DForOutWhenUnconnected=off
  wires:
  Demux1/4 -> BusCreator1/4  "MCU MotorIn1 rotv"
  Demux1/10 -> BusCreator1/10  "MCU MotorIn1 Current_u"
  BusCreator1/1 -> Out/1
  Demux1/7 -> BusCreator1/7  "MCU MotorIn1 VoltBatt"
  Demux1/8 -> BusCreator1/8  "MCU MotorIn1 Current_d"
  Demux1/1 -> BusCreator1/1  "MCU MotorIn1 Trq_trg"
  Demux1/9 -> BusCreator1/9  "MCU MotorIn1 Current_q"
  Demux1/5 -> BusCreator1/5  "MCU MotorIn1 rot"
  In/1 -> Demux1/1
  Demux1/2 -> BusCreator1/2  "MCU MotorIn1 Trq"
  Demux1/3 -> BusCreator1/3  "MCU MotorIn1 rotv_trg"
  Demux1/6 -> BusCreator1/6  "MCU MotorIn1 PwrElec"
  Demux1/12 -> BusCreator1/12  "MCU MotorIn1 Current_w"
  Demux1/11 -> BusCreator1/11  "MCU MotorIn1 Current_v"

== system generic_src/CarMaker/IPG Vehicle/PowerTrain/MCU Example/PTMotorCU_In/CreateBus MCU MotorIn2 ==
  In : Inport
  BusCreator1 : BusCreator  Inputs=12
  Demux1 : Demux  Outputs=12
      settings: DisplayOption=none
  Out : Outport  VectorParamsAs1DForOutWhenUnconnected=off
  wires:
  Demux1/1 -> BusCreator1/1  "MCU MotorIn2 Trq_trg"
  Demux1/5 -> BusCreator1/5  "MCU MotorIn2 rot"
  BusCreator1/1 -> Out/1
  Demux1/9 -> BusCreator1/9  "MCU MotorIn2 Current_q"
  Demux1/3 -> BusCreator1/3  "MCU MotorIn2 rotv_trg"
  Demux1/4 -> BusCreator1/4  "MCU MotorIn2 rotv"
  Demux1/7 -> BusCreator1/7  "MCU MotorIn2 VoltBatt"
  Demux1/12 -> BusCreator1/12  "MCU MotorIn2 Current_w"
  In/1 -> Demux1/1
  Demux1/2 -> BusCreator1/2  "MCU MotorIn2 Trq"
  Demux1/8 -> BusCreator1/8  "MCU MotorIn2 Current_d"
  Demux1/11 -> BusCreator1/11  "MCU MotorIn2 Current_v"
  Demux1/6 -> BusCreator1/6  "MCU MotorIn2 PwrElec"
  Demux1/10 -> BusCreator1/10  "MCU MotorIn2 Current_u"

== system generic_src/CarMaker/IPG Vehicle/PowerTrain/MCU Example/PTMotorCU_In/CreateBus MCU MotorIn3 ==
  In : Inport
  BusCreator1 : BusCreator  Inputs=12
  Demux1 : Demux  Outputs=12
      settings: DisplayOption=none
  Out : Outport  VectorParamsAs1DForOutWhenUnconnected=off
  wires:
  BusCreator1/1 -> Out/1
  Demux1/5 -> BusCreator1/5  "MCU MotorIn3 rot"
  Demux1/7 -> BusCreator1/7  "MCU MotorIn3 VoltBatt"
  Demux1/6 -> BusCreator1/6  "MCU MotorIn3 PwrElec"
  Demux1/8 -> BusCreator1/8  "MCU MotorIn3 Current_d"
  Demux1/9 -> BusCreator1/9  "MCU MotorIn3 Current_q"
  Demux1/11 -> BusCreator1/11  "MCU MotorIn3 Current_v"
  Demux1/1 -> BusCreator1/1  "MCU MotorIn3 Trq_trg"
  Demux1/10 -> BusCreator1/10  "MCU MotorIn3 Current_u"
  Demux1/4 -> BusCreator1/4  "MCU MotorIn3 rotv"
  Demux1/12 -> BusCreator1/12  "MCU MotorIn3 Current_w"
  Demux1/2 -> BusCreator1/2  "MCU MotorIn3 Trq"
  In/1 -> Demux1/1
  Demux1/3 -> BusCreator1/3  "MCU MotorIn3 rotv_trg"

== system generic_src/CarMaker/IPG Vehicle/PowerTrain/MCU Example/PTMotorCU_In/CreateBus MCU MotorOut0 ==
  In : Inport
  BusCreator : BusCreator  Inputs=1
  Demux : Demux  Outputs=1
      settings: DisplayOption=none
  Out : Outport  VectorParamsAs1DForOutWhenUnconnected=off
  wires:
  Demux/1 -> BusCreator/1  "MCU MotorOut0 Load"
  BusCreator/1 -> Out/1
  In/1 -> Demux/1

== system generic_src/CarMaker/IPG Vehicle/PowerTrain/MCU Example/PTMotorCU_In/CreateBus MCU MotorOut1 ==
  In : Inport
  BusCreator : BusCreator  Inputs=1
  Demux : Demux  Outputs=1
      settings: DisplayOption=none
  Out : Outport  VectorParamsAs1DForOutWhenUnconnected=off
  wires:
  Demux/1 -> BusCreator/1  "MCU MotorOut1 Load"
  In/1 -> Demux/1
  BusCreator/1 -> Out/1

== system generic_src/CarMaker/IPG Vehicle/PowerTrain/MCU Example/PTMotorCU_In/CreateBus MCU MotorOut2 ==
  In : Inport
  BusCreator : BusCreator  Inputs=1
  Demux : Demux  Outputs=1
      settings: DisplayOption=none
  Out : Outport  VectorParamsAs1DForOutWhenUnconnected=off
  wires:
  Demux/1 -> BusCreator/1  "MCU MotorOut2 Load"
  BusCreator/1 -> Out/1
  In/1 -> Demux/1

== system generic_src/CarMaker/IPG Vehicle/PowerTrain/MCU Example/PTMotorCU_In/CreateBus MCU MotorOut3 ==
  In : Inport
  BusCreator : BusCreator  Inputs=1
  Demux : Demux  Outputs=1
      settings: DisplayOption=none
  Out : Outport  VectorParamsAs1DForOutWhenUnconnected=off
  wires:
  Demux/1 -> BusCreator/1  "MCU MotorOut3 Load"
  BusCreator/1 -> Out/1
  In/1 -> Demux/1

== system generic_src/CarMaker/IPG Vehicle/PowerTrain/MCU Example/PTMotorCU_In/CreateBus MCU_Cfg ISG ==
  In : Inport
  BusCreator : BusCreator  Inputs=4
  Demux : Demux
      settings: DisplayOption=none
  Out : Outport  VectorParamsAs1DForOutWhenUnconnected=off
  wires:
  Demux/3 -> BusCreator/3  "MCU_Cfg ISG rotv_Mot_max"
  Demux/2 -> BusCreator/2  "MCU_Cfg ISG Ratio"
  Demux/4 -> BusCreator/4  "MCU_Cfg ISG rotv_Gen_max"
  BusCreator/1 -> Out/1
  Demux/1 -> BusCreator/1  "MCU_Cfg ISG CtrlMode"
  In/1 -> Demux/1

== system generic_src/CarMaker/IPG Vehicle/PowerTrain/MCU Example/PTMotorCU_In/CreateBus MCU_Cfg Misc ==
  In : Inport
  BusCreator : BusCreator  Inputs=1
  Demux : Demux  Outputs=1
      settings: DisplayOption=none
  Out : Outport  VectorParamsAs1DForOutWhenUnconnected=off
  wires:
  Demux/1 -> BusCreator/1  "MCU_Cfg nMotor"
  BusCreator/1 -> Out/1
  In/1 -> Demux/1

== system generic_src/CarMaker/IPG Vehicle/PowerTrain/MCU Example/PTMotorCU_In/CreateBus MCU_Cfg Motor0 ==
  In : Inport
  BusCreator1 : BusCreator  Inputs=4
  Demux1 : Demux
      settings: DisplayOption=none
  Out : Outport  VectorParamsAs1DForOutWhenUnconnected=off
  wires:
  Demux1/4 -> BusCreator1/4  "MCU_Cfg Motor0 rotv_Gen_max"
  Demux1/2 -> BusCreator1/2  "MCU_Cfg Motor0 Ratio"
  Demux1/3 -> BusCreator1/3  "MCU_Cfg Motor0 rotv_Mot_max"
  Demux1/1 -> BusCreator1/1  "MCU_Cfg Motor0 CtrlMode"
  In/1 -> Demux1/1
  BusCreator1/1 -> Out/1

== system generic_src/CarMaker/IPG Vehicle/PowerTrain/MCU Example/PTMotorCU_In/CreateBus MCU_Cfg Motor1 ==
  In : Inport
  BusCreator : BusCreator  Inputs=4
  Demux : Demux
      settings: DisplayOption=none
  Out : Outport  VectorParamsAs1DForOutWhenUnconnected=off
  wires:
  Demux/4 -> BusCreator/4  "MCU_Cfg Motor1 rotv_Gen_max"
  Demux/2 -> BusCreator/2  "MCU_Cfg Motor1 Ratio"
  Demux/3 -> BusCreator/3  "MCU_Cfg Motor1 rotv_Mot_max"
  Demux/1 -> BusCreator/1  "MCU_Cfg Motor1 CtrlMode"
  In/1 -> Demux/1
  BusCreator/1 -> Out/1

== system generic_src/CarMaker/IPG Vehicle/PowerTrain/MCU Example/PTMotorCU_In/CreateBus MCU_Cfg Motor2 ==
  In : Inport
  BusCreator : BusCreator  Inputs=4
  Demux : Demux
      settings: DisplayOption=none
  Out : Outport  VectorParamsAs1DForOutWhenUnconnected=off
  wires:
  Demux/4 -> BusCreator/4  "MCU_Cfg Motor2 rotv_Gen_max"
  Demux/1 -> BusCreator/1  "MCU_Cfg Motor2 CtrlMode"
  Demux/2 -> BusCreator/2  "MCU_Cfg Motor2 Ratio"
  Demux/3 -> BusCreator/3  "MCU_Cfg Motor2 rotv_Mot_max"
  BusCreator/1 -> Out/1
  In/1 -> Demux/1

== system generic_src/CarMaker/IPG Vehicle/PowerTrain/MCU Example/PTMotorCU_In/CreateBus MCU_Cfg Motor3 ==
  In : Inport
  BusCreator : BusCreator  Inputs=4
  Demux : Demux
      settings: DisplayOption=none
  Out : Outport  VectorParamsAs1DForOutWhenUnconnected=off
  wires:
  Demux/4 -> BusCreator/4  "MCU_Cfg Motor3 rotv_Gen_max"
  Demux/1 -> BusCreator/1  "MCU_Cfg Motor3 CtrlMode"
  Demux/2 -> BusCreator/2  "MCU_Cfg Motor3 Ratio"
  Demux/3 -> BusCreator/3  "MCU_Cfg Motor3 rotv_Mot_max"
  BusCreator/1 -> Out/1
  In/1 -> Demux/1

== system generic_src/CarMaker/IPG Vehicle/PowerTrain/MCU Example/PTMotorCU_Out/Adapt MCU ISGOut from CM12 to CM13 ==
  In : Inport
  Demux : Demux  Outputs=5
  Ground : Ground
  Mux : Mux  Inputs=6
  Out : Outport
  wires:
  Demux/5 -> Mux/6  "MCU ISGOut Voltage_w"
  Ground/1 -> Demux/1
  In/1 -> Mux/1
  Mux/1 -> Out/1
  Demux/4 -> Mux/5  "MCU ISGOut Voltage_v"
  Demux/1 -> Mux/2  "MCU ISGOut Voltage_d"
  Demux/3 -> Mux/4  "MCU ISGOut Voltage_u"
  Demux/2 -> Mux/3  "MCU ISGOut Voltage_q"

== system generic_src/CarMaker/IPG Vehicle/PowerTrain/MCU Example/PTMotorCU_Out/Adapt MCU MotorOut0 from CM12 to CM13 ==
  In : Inport
  Demux : Demux  Outputs=5
  Ground : Ground
  Mux : Mux  Inputs=6
  Out : Outport
  wires:
  Demux/2 -> Mux/3  "MCU MotorOut0 Voltage_q"
  Demux/3 -> Mux/4  "MCU MotorOut0 Voltage_u"
  Demux/1 -> Mux/2  "MCU MotorOut0 Voltage_d"
  Demux/4 -> Mux/5  "MCU MotorOut0 Voltage_v"
  Mux/1 -> Out/1
  In/1 -> Mux/1
  Ground/1 -> Demux/1
  Demux/5 -> Mux/6  "MCU MotorOut0 Voltage_w"

== system generic_src/CarMaker/IPG Vehicle/PowerTrain/MCU Example/PTMotorCU_Out/Adapt MCU MotorOut1 from CM12 to CM13 ==
  In : Inport
  Demux : Demux  Outputs=5
  Ground : Ground
  Mux : Mux  Inputs=6
  Out : Outport
  wires:
  Demux/5 -> Mux/6  "MCU MotorOut1 Voltage_w"
  Ground/1 -> Demux/1
  In/1 -> Mux/1
  Mux/1 -> Out/1
  Demux/4 -> Mux/5  "MCU MotorOut1 Voltage_v"
  Demux/1 -> Mux/2  "MCU MotorOut1 Voltage_d"
  Demux/3 -> Mux/4  "MCU MotorOut1 Voltage_u"
  Demux/2 -> Mux/3  "MCU MotorOut1 Voltage_q"

== system generic_src/CarMaker/IPG Vehicle/PowerTrain/MCU Example/PTMotorCU_Out/Adapt MCU MotorOut2 from CM12 to CM13 ==
  In : Inport
  Demux : Demux  Outputs=5
  Ground : Ground
  Mux : Mux  Inputs=6
  Out : Outport
  wires:
  Demux/2 -> Mux/3  "MCU MotorOut2 Voltage_q"
  Demux/3 -> Mux/4  "MCU MotorOut2 Voltage_u"
  Demux/1 -> Mux/2  "MCU MotorOut2 Voltage_d"
  Demux/4 -> Mux/5  "MCU MotorOut2 Voltage_v"
  Mux/1 -> Out/1
  In/1 -> Mux/1
  Ground/1 -> Demux/1
  Demux/5 -> Mux/6  "MCU MotorOut2 Voltage_w"

== system generic_src/CarMaker/IPG Vehicle/PowerTrain/MCU Example/PTMotorCU_Out/Adapt MCU MotorOut3 from CM12 to CM13 ==
  In : Inport
  Demux : Demux  Outputs=5
  Ground : Ground
  Mux : Mux  Inputs=6
  Out : Outport
  wires:
  Demux/5 -> Mux/6  "MCU MotorOut3 Voltage_w"
  Ground/1 -> Demux/1
  In/1 -> Mux/1
  Mux/1 -> Out/1
  Demux/4 -> Mux/5  "MCU MotorOut3 Voltage_v"
  Demux/1 -> Mux/2  "MCU MotorOut3 Voltage_d"
  Demux/3 -> Mux/4  "MCU MotorOut3 Voltage_u"
  Demux/2 -> Mux/3  "MCU MotorOut3 Voltage_q"

== system generic_src/CarMaker/IPG Vehicle/PowerTrain/PTControl Example/PTC ClutchOut/CreateBus PTC ClutchOut0 ==
  In : Inport
  BusCreator : BusCreator  Inputs=3
  Demux : Demux  Outputs=3
      settings: DisplayOption=none
  Out : Outport  VectorParamsAs1DForOutWhenUnconnected=off
  wires:
  Demux/3 -> BusCreator/3  "PTC ClutchOut0 Trq_out_trg"
  Demux/2 -> BusCreator/2  "PTC ClutchOut0 rotv_out_trg"
  Demux/1 -> BusCreator/1  "PTC ClutchOut0 Pos"
  BusCreator/1 -> Out/1
  In/1 -> Demux/1

== system generic_src/CarMaker/IPG Vehicle/PowerTrain/PTControl Example/PTC ClutchOut/CreateBus PTC ClutchOut1 ==
  In : Inport
  BusCreator : BusCreator  Inputs=3
  Demux : Demux  Outputs=3
      settings: DisplayOption=none
  Out : Outport  VectorParamsAs1DForOutWhenUnconnected=off
  wires:
  Demux/3 -> BusCreator/3  "PTC ClutchOut1 Trq_out_trg"
  Demux/2 -> BusCreator/2  "PTC ClutchOut1 rotv_out_trg"
  Demux/1 -> BusCreator/1  "PTC ClutchOut1 Pos"
  BusCreator/1 -> Out/1
  In/1 -> Demux/1

== system generic_src/CarMaker/IPG Vehicle/PowerTrain/PTControl Example/PTC ClutchOut/CreateBus PTC ClutchOut10 ==
  In : Inport
  BusCreator : BusCreator  Inputs=3
  Demux : Demux  Outputs=3
      settings: DisplayOption=none
  Out : Outport  VectorParamsAs1DForOutWhenUnconnected=off
  wires:
  Demux/3 -> BusCreator/3  "PTC ClutchOut10 Trq_out_trg"
  Demux/2 -> BusCreator/2  "PTC ClutchOut10 rotv_out_trg"
  Demux/1 -> BusCreator/1  "PTC ClutchOut10 Pos"
  BusCreator/1 -> Out/1
  In/1 -> Demux/1

== system generic_src/CarMaker/IPG Vehicle/PowerTrain/PTControl Example/PTC ClutchOut/CreateBus PTC ClutchOut11 ==
  In : Inport
  BusCreator : BusCreator  Inputs=3
  Demux : Demux  Outputs=3
      settings: DisplayOption=none
  Out : Outport  VectorParamsAs1DForOutWhenUnconnected=off
  wires:
  Demux/3 -> BusCreator/3  "PTC ClutchOut11 Trq_out_trg"
  Demux/2 -> BusCreator/2  "PTC ClutchOut11 rotv_out_trg"
  Demux/1 -> BusCreator/1  "PTC ClutchOut11 Pos"
  BusCreator/1 -> Out/1
  In/1 -> Demux/1
